simulink model "trabalho_funcionando"  (R2015a)
settings: Solver=ode23t  StartTime=0.0  StopTime=0.6  RelTol=1e-3
libraries: fl_lib x33, elec_lib x22, nesl_utility x22
Description:
  | Low-Noise Bipolar Transistor Voltage Amplifier
  | 
  | This example shows a typical low-noise audio amplifier circuit.
  | Resistor R2 provides negative feedback to stabilize the overall
  | amplifier gain, making it independent of transistor open-loop
  | forward transfer gain. Circuit gain is approximately defined by
  | (R1+R2)/R1 = 101. The simulation shows that it takes the circuit
  | a few seconds to settle to its steady operating point, and that the
  | output is initially clipped. Input u and output y are included to
  | support linearization.
  | 
  | If you have Simulink(R) Control Design(TM) installed, then to plot the
  | frequency response, select Analysis->Control Design-> Linear
  | Analysis to open the Linear Analysis Tool.
  | Before linearizing, you need to select the Solver Configuration block
  | option "Start simulation from steady state" to ensure that the model
  | is linearized about its nominal operating point. Change the Plot
  | Result to New Bode, and then click on Linearize. The linearization
  | points are defined by right-clicking on a Simulink(R) line, and
  | selecting Linearization Points.
  | If you look at the measurement block with input port V1, you will see
  | the linearization output symbol at the output of the PS-Simulink(R)
  | block. Similarly under the Source block you will see a linearization
  | input point symbol on the output of the Sine Wave block.
  | 
  | If you do not have Simulink Control Design, then you can
  | linearize the model between input port u and output port y
  | by typing:
  | 
  | [a,b,c,d] = linmod('elec_bipolar_low_noise_amp')
  | 
  | The frequency response can then be plotted using the
  | Control System Toolbox(TM) by typing:
  | 
  | bode(a,b,c,d)
  | 
  | 
  | 
  | Copyright 2008-2015 The MathWorks, Inc.
settings Model: CovSFcnEnable=off  Creator=MathWorks  LastModifiedBy=João Pedro
settings DataIOCC: SignalLoggingSaveFormat=ModelDataLogs
settings OptimizationCC: ExpressionDepthLimit=2147483647
settings DebuggingCC: UnderspecifiedInitializationDetection=Classic  MergeDetectMultiDrivingBlocksExec=none  FcnCallInpInsideContextMsg=UseLocalSettings  StateNameClashWarn=warning
settings GRTTargetCC: CombineOutputUpdateFcns=off  GRTInterface=on

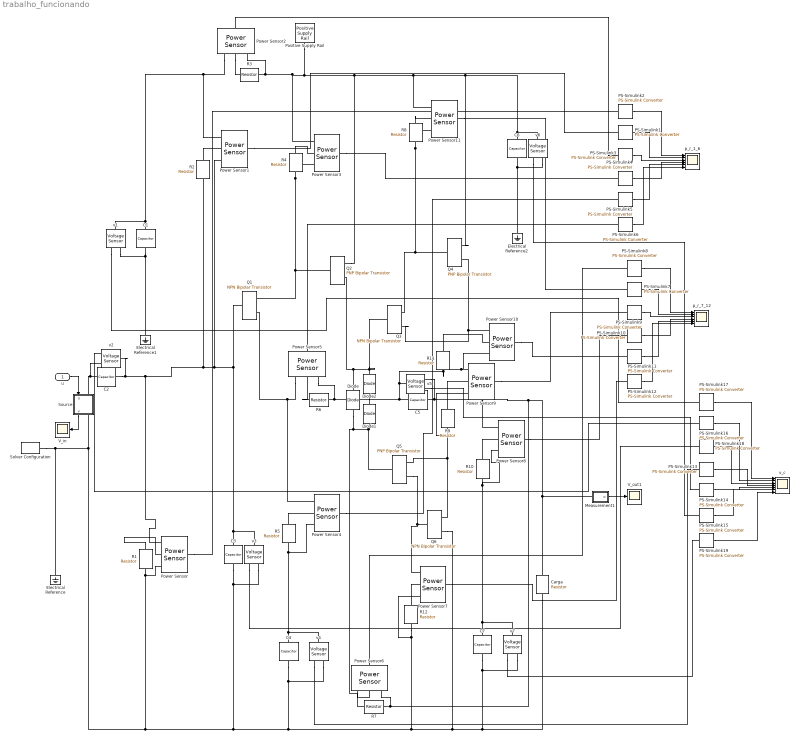
== system trabalho_funcionando ==
  u : Inport
  C1 : fl_lib/Electrical/Electrical Elements/Capacitor  c=2.2 uF  r=10 Ohm  g=0 1/Ohm  i_specify=off  i_priority=High  i=0 A  v_specify=off  v_priority=High  v=0 V  vc_specify=on  vc_priority=High  vc=0 V
  C2 : fl_lib/Electrical/Electrical Elements/Capacitor  c=1 uF  r=10 Ohm  g=0 1/Ohm  i_specify=off  i_priority=High  i=0 A  v_specify=off  v_priority=High  v=0 V  vc_specify=on  vc_priority=High  vc=0 V
  C3 : fl_lib/Electrical/Electrical Elements/Capacitor  c=47 pF  r=0.1 Ohm  g=0 1/Ohm  i_specify=off  i_priority=High  i=0 A  v_specify=off  v_priority=High  v=0 V  vc_specify=on  vc_priority=High  vc=0 V
  C4 : fl_lib/Electrical/Electrical Elements/Capacitor  c=47 uF  r=0.1 Ohm  g=0 1/Ohm  i_specify=off  i_priority=High  i=0 A  v_specify=off  v_priority=High  v=0 V  vc_specify=on  vc_priority=High  vc=0 V
  C5 : fl_lib/Electrical/Electrical Elements/Capacitor  c=2200 uF  r=0.1 Ohm  g=0 1/Ohm  i_specify=off  i_priority=High  i=0 A  v_specify=off  v_priority=High  v=0 V  vc_specify=on  vc_priority=High  vc=0 V
  C6 : fl_lib/Electrical/Electrical Elements/Capacitor  c=0.1 uF  r=10 Ohm  g=0 1/Ohm  i_specify=off  i_priority=High  i=0 A  v_specify=off  v_priority=High  v=0 V  vc_specify=on  vc_priority=High  vc=0 V
  C7 : fl_lib/Electrical/Electrical Elements/Capacitor  c=0.1 uF  r=10 Ohm  g=0 1/Ohm  i_specify=off  i_priority=High  i=0 A  v_specify=off  v_priority=High  v=0 V  vc_specify=on  vc_priority=High  vc=0 V
  Carga : fl_lib/Electrical/Electrical Elements/Resistor  R=4 Ohm  i_specify=off  i_priority=High  i=0 A  v_specify=off  v_priority=High  v=0 V
  Diode : elec_lib/Semiconductor Devices/Diode  ModelType=1  Vf=0.1 V  Ron=0.3 Ohm  Goff=1e-8 S  Rz=0.3 Ohm  Vz=50 V  C_PWL=5 pF  prmExp=1  I12=[ 0.0137 0.545 ] A  V12=[ 0.6 0.7 ] V  I1=0.0137 A  V1=0.6 V  RS=0.01 Ohm  IS=1e-12 A  Tmeas=25 C  ec=1  BV=Inf V  C_param=1  CJ0=5 pF  VJ=1 V  Mgrad=0.5  Vvec=[ 0.1 10 100 ] V  Cvec=[ 3.5 1 0.4 ] pF  FC=0.5  Q_param=1  Irrm=-7.15 A  iF=4 A  didt=-750 A/us  trr=115 ns  TT=50 ns  tau=100 ns  T_param=1  IS_T2=1.25e-7 A  I1_T2=0.245 A  V1_T2=0.5 V  Tmeas2=125 C  EG_param=1  EG=1.11 eV  XTI_param=1  XTI=3  dBVdT=0 V/K  Tdevice=25 C  Rth=[ 0 10 ] K/W  thermal_mass_parameterization=1  thermal_mass=[ 0 1 ] J/K  thermal_time_constant=[ 0 10 ] s  thermal_mass_initial_temperatures=[ 25 25 ] C
  Diode1 : elec_lib/Semiconductor Devices/Diode  ModelType=1  Vf=0.1 V  Ron=0.3 Ohm  Goff=1e-8 S  Rz=0.3 Ohm  Vz=50 V  C_PWL=5 pF  prmExp=1  I12=[ 0.0137 0.545 ] A  V12=[ 0.6 0.7 ] V  I1=0.0137 A  V1=0.6 V  RS=0.01 Ohm  IS=1e-12 A  Tmeas=25 C  ec=1  BV=Inf V  C_param=1  CJ0=5 pF  VJ=1 V  Mgrad=0.5  Vvec=[ 0.1 10 100 ] V  Cvec=[ 3.5 1 0.4 ] pF  FC=0.5  Q_param=1  Irrm=-7.15 A  iF=4 A  didt=-750 A/us  trr=115 ns  TT=50 ns  tau=100 ns  T_param=1  IS_T2=1.25e-7 A  I1_T2=0.245 A  V1_T2=0.5 V  Tmeas2=125 C  EG_param=1  EG=1.11 eV  XTI_param=1  XTI=3  dBVdT=0 V/K  Tdevice=25 C  Rth=[ 0 10 ] K/W  thermal_mass_parameterization=1  thermal_mass=[ 0 1 ] J/K  thermal_time_constant=[ 0 10 ] s  thermal_mass_initial_temperatures=[ 25 25 ] C
  Diode2 : elec_lib/Semiconductor Devices/Diode  ModelType=1  Vf=0.1 V  Ron=0.3 Ohm  Goff=1e-8 S  Rz=0.3 Ohm  Vz=50 V  C_PWL=5 pF  prmExp=1  I12=[ 0.0137 0.545 ] A  V12=[ 0.6 0.7 ] V  I1=0.0137 A  V1=0.6 V  RS=0.01 Ohm  IS=1e-12 A  Tmeas=25 C  ec=1  BV=Inf V  C_param=1  CJ0=5 pF  VJ=1 V  Mgrad=0.5  Vvec=[ 0.1 10 100 ] V  Cvec=[ 3.5 1 0.4 ] pF  FC=0.5  Q_param=1  Irrm=-7.15 A  iF=4 A  didt=-750 A/us  trr=115 ns  TT=50 ns  tau=100 ns  T_param=1  IS_T2=1.25e-7 A  I1_T2=0.245 A  V1_T2=0.5 V  Tmeas2=125 C  EG_param=1  EG=1.11 eV  XTI_param=1  XTI=3  dBVdT=0 V/K  Tdevice=25 C  Rth=[ 0 10 ] K/W  thermal_mass_parameterization=1  thermal_mass=[ 0 1 ] J/K  thermal_time_constant=[ 0 10 ] s  thermal_mass_initial_temperatures=[ 25 25 ] C
  Electrical Reference : fl_lib/Electrical/Electrical Elements/Electrical Reference
  Electrical Reference1 : fl_lib/Electrical/Electrical Elements/Electrical Reference
  Electrical Reference2 : fl_lib/Electrical/Electrical Elements/Electrical Reference
  Measurement1 : Subsystem
  PS-Simulink{1..19} (19 alike) : nesl_utility/PS-Simulink Converter  PhysicalDomain=network_engine_domain  SubClassName=ps_output  LeftPortType=input  RightPortType=output  PseudoPeriodic=off  Frequencies=[]  Unit=1  AffineConversion=off
  Positive Supply Rail : elec_lib/Sources/Positive Supply Rail  v0=54 V
  Power Sensor{,1..11} (12 alike) : elec_lib/Sensors/Power Sensor  measurement_type=1  averaging_period=1e-4 s
  Q1 : elec_lib/Semiconductor Devices/NPN Bipolar Transistor  parameterization=2  prmDatasheet=1  prmEquCoeff=1  BF=458.7  IS=4.68e-14 A  ec=1  VAF=52.64 V  hfe=520  hoe=5e-05 1/Ohm  Ic_h=100 mA  Vce_h=5 V  V1=0.55 V  I1=0.5 mA  BR=11.57  Tmeas=25 C  RC=1 Ohm  RE=0.26 Ohm  RB=1 Ohm  C_BC=4 pF  C_BE=4 pF  TF=0 us  TR=0 us  hfe_T2=125  XTB=0  V1_T2=0.45 V  I1_T2=0.5 mA  Tmeas2=125 C  EG=1.11 eV  XTI=3  TdeviceDatasheet=25 C  TdeviceEquCoeff=25 C  Rth=[ 0 10 ] K/W  thermal_mass_parameterization=1  thermal_mass=[ 0 1 ] J/K  thermal_time_constant=[ 0 10 ] s  thermal_mass_initial_temperatures=[ 25 25 ] C
  Q2 : elec_lib/Semiconductor Devices/PNP Bipolar Transistor  parameterization=2  prmDatasheet=1  prmEquCoeff=1  BF=449.8  IS=2.077e-13 A  ec=1  VAF=29 V  hfe=100  hoe=5e-5 1/Ohm  Ic_h=-1 mA  Vce_h=-5 V  V1=-0.55 V  I1=-0.5 mA  BR=20.92  Tmeas=25 C  RC=0.32 Ohm  RE=0.14 Ohm  RB=40 Ohm  C_BC=5 pF  C_BE=5 pF  TF=0 us  TR=0 us  hfe_T2=125  XTB=0  V1_T2=-0.45 V  I1_T2=-0.5 mA  Tmeas2=125 C  EG=1.11 eV  XTI=3  TdeviceDatasheet=25 C  TdeviceEquCoeff=25 C  Rth=[ 0 10 ] K/W  thermal_mass_parameterization=1  thermal_mass=[ 0 1 ] J/K  thermal_time_constant=[ 0 10 ] s  thermal_mass_initial_temperatures=[ 25 25 ] C
  Q3 : elec_lib/Semiconductor Devices/NPN Bipolar Transistor  parameterization=2  prmDatasheet=1  prmEquCoeff=1  BF=153.42  IS=800e-15 A  ec=1  VAF=4.8443 V  hfe=100  hoe=5e-05 1/Ohm  Ic_h=1 mA  Vce_h=5 V  V1=0.55 V  I1=0.5 mA  BR=39.462  Tmeas=25 C  RC=39.911 Ohm  RE=0.005 Ohm  RB=0.574 Ohm  C_BC=4 pF  C_BE=4 pF  TF=0 us  TR=0 us  hfe_T2=125  XTB=0  V1_T2=0.45 V  I1_T2=0.5 mA  Tmeas2=125 C  EG=1.11 eV  XTI=3  TdeviceDatasheet=25 C  TdeviceEquCoeff=25 C  Rth=[ 0 10 ] K/W  thermal_mass_parameterization=1  thermal_mass=[ 0 1 ] J/K  thermal_time_constant=[ 0 10 ] s  thermal_mass_initial_temperatures=[ 25 25 ] C
  Q4 : elec_lib/Semiconductor Devices/PNP Bipolar Transistor  parameterization=2  prmDatasheet=1  prmEquCoeff=1  BF=65.974  IS=7.899e-11 A  ec=1  VAF=10.7084 V  hfe=100  hoe=5e-5 1/Ohm  Ic_h=-1 mA  Vce_h=-5 V  V1=-0.55 V  I1=-0.5 mA  BR=1.9619  Tmeas=25 C  RC=0.12 Ohm  RE=1e-4 Ohm  RB=2.355 Ohm  C_BC=5 pF  C_BE=5 pF  TF=0 us  TR=0 us  hfe_T2=125  XTB=0  V1_T2=-0.45 V  I1_T2=-0.5 mA  Tmeas2=125 C  EG=1.11 eV  XTI=3  TdeviceDatasheet=25 C  TdeviceEquCoeff=25 C  Rth=[ 0 10 ] K/W  thermal_mass_parameterization=1  thermal_mass=[ 0 1 ] J/K  thermal_time_constant=[ 0 10 ] s  thermal_mass_initial_temperatures=[ 25 25 ] C
  Q5 : elec_lib/Semiconductor Devices/PNP Bipolar Transistor  parameterization=2  prmDatasheet=1  prmEquCoeff=1  BF=222.84  IS=400e-15 A  ec=1  VAF=30.600 V  hfe=100  hoe=5e-5 1/Ohm  Ic_h=-1 mA  Vce_h=-5 V  V1=-0.55 V  I1=-0.5 mA  BR=10.181  Tmeas=25 C  RC=0.27337 Ohm  RE=40e-3 Ohm  RB=1.7344 Ohm  C_BC=5 pF  C_BE=5 pF  TF=0 us  TR=0 us  hfe_T2=125  XTB=0  V1_T2=-0.45 V  I1_T2=-0.5 mA  Tmeas2=125 C  EG=1.11 eV  XTI=3  TdeviceDatasheet=25 C  TdeviceEquCoeff=25 C  Rth=[ 0 10 ] K/W  thermal_mass_parameterization=1  thermal_mass=[ 0 1 ] J/K  thermal_time_constant=[ 0 10 ] s  thermal_mass_initial_temperatures=[ 25 25 ] C
  Q6 : elec_lib/Semiconductor Devices/NPN Bipolar Transistor  parameterization=2  prmDatasheet=1  prmEquCoeff=1  BF=73  IS=2.37e-8 A  ec=1  VAF=100 V  hfe=100  hoe=5e-05 1/Ohm  Ic_h=1 mA  Vce_h=5 V  V1=0.55 V  I1=0.5 mA  BR=2.66  Tmeas=25 C  RC=0.0856 Ohm  RE=0.000856 Ohm  RB=0.81 Ohm  C_BC=4 pF  C_BE=4 pF  TF=0 us  TR=0 us  hfe_T2=125  XTB=0  V1_T2=0.45 V  I1_T2=0.5 mA  Tmeas2=125 C  EG=1.11 eV  XTI=3  TdeviceDatasheet=25 C  TdeviceEquCoeff=25 C  Rth=[ 0 10 ] K/W  thermal_mass_parameterization=1  thermal_mass=[ 0 1 ] J/K  thermal_time_constant=[ 0 10 ] s  thermal_mass_initial_temperatures=[ 25 25 ] C
  R1 : fl_lib/Electrical/Electrical Elements/Resistor  R=220 kOhm  i_specify=off  i_priority=High  i=0 A  v_specify=off  v_priority=High  v=0 V
  R10 : fl_lib/Electrical/Electrical Elements/Resistor  R=10 Ohm  i_specify=off  i_priority=High  i=0 A  v_specify=off  v_priority=High  v=0 V
  R11 : fl_lib/Electrical/Electrical Elements/Resistor  R=0.47 Ohm  i_specify=off  i_priority=High  i=0 A  v_specify=off  v_priority=High  v=0 V
  R12 : fl_lib/Electrical/Electrical Elements/Resistor  R=180 Ohm  i_specify=off  i_priority=High  i=0 A  v_specify=off  v_priority=High  v=0 V
  R2 : fl_lib/Electrical/Electrical Elements/Resistor  R=150 kOhm  i_specify=off  i_priority=High  i=0 A  v_specify=off  v_priority=High  v=0 V
  R3 : fl_lib/Electrical/Electrical Elements/Resistor  R=47 kOhm  i_specify=off  i_priority=High  i=0 A  v_specify=off  v_priority=High  v=0 V
  R4 : fl_lib/Electrical/Electrical Elements/Resistor  R=5.6 kOhm  i_specify=off  i_priority=High  i=0 A  v_specify=off  v_priority=High  v=0 V
  R5 : fl_lib/Electrical/Electrical Elements/Resistor  R=270 Ohm  i_specify=off  i_priority=High  i=0 A  v_specify=off  v_priority=High  v=0 V
  R6 : fl_lib/Electrical/Electrical Elements/Resistor  R=10 kOhm  i_specify=off  i_priority=High  i=0 A  v_specify=off  v_priority=High  v=0 V
  R7 : fl_lib/Electrical/Electrical Elements/Resistor  R=8.2 kOhm  i_specify=off  i_priority=High  i=0 A  v_specify=off  v_priority=High  v=0 V
  R8 : fl_lib/Electrical/Electrical Elements/Resistor  R=180 Ohm  i_specify=off  i_priority=High  i=0 A  v_specify=off  v_priority=High  v=0 V
  R9 : fl_lib/Electrical/Electrical Elements/Resistor  R=0.39 Ohm  i_specify=off  i_priority=High  i=0 A  v_specify=off  v_priority=High  v=0 V
  Solver Configuration : nesl_utility/Solver Configuration  PhysicalDomain=network_engine_domain  SubClassName=solver  LeftPortType=input  RightPortType=generic  Accelerate=off  Tones=[]  Harmonics=[]  SimulateNoise=off  Profile=off  UseLocalSampling=off  EnableSwitchedLinearOptims=on  FrequencyDomain=off  UseCCode=off  RelTol=0.001  AbsTol=1e-06  MinStep=1e-09  ToWorkspace=off  RevertToSquareIcSolve=off  NumHomotopyIterations=100  DoDC=off  ResidualTolerance=1e-9  UseLocalSolver=off  LocalSolverChoice=NE_BACKWARD_EULER_ADVANCER  LocalSolverSampleTime=1e-5  DoFixedCost=off  MaxNonlinIter=2  MaxModeIter=2  LinearAlgebra=Sparse  DelaysMemoryBudget=1024  AutomaticFiltering=on  FilteringTimeConstant=0.001
  Source : Subsystem
  V_in : Scope
      settings: TimeRange=0.01  YMin=-0.1  YMax=0.1
  V_out1 : Scope
      settings: TimeRange=0.01  YMin=-10  YMax=10  SaveName=ScopeData2
  p_r_1_6 : Scope  NumInputPorts=6
      settings: TimeRange=0.01  YMin=-10~-5~-5~-5~-5~-5  YMax=10~5~5~5~5~5
  p_r_7_12 : Scope  NumInputPorts=6
      settings: TimeRange=0.01  YMin=-10~-5~-5~-5~-5~-5  YMax=10~5~5~5~5~5  SaveName=ScopeData3
  v{1..7} (7 alike) : fl_lib/Electrical/Electrical Sensors/Voltage Sensor
  v_c : Scope  NumInputPorts=7
      settings: TimeRange=0.01  YMin=-10~-5~-5~-5~-5~-5~-5  YMax=10~5~5~5~5~5~5  SaveName=ScopeData4
  wires:
  Source/1(v) -> V_in/1
  u/1 -> Source/1(u)
  Measurement1/1(o) -> V_out1/1
  PS-Simulink2/1 -> p_r_1_6/1
  PS-Simulink1/1 -> p_r_1_6/2
  PS-Simulink3/1 -> p_r_1_6/3
  PS-Simulink4/1 -> p_r_1_6/4
  PS-Simulink5/1 -> p_r_1_6/5
  PS-Simulink6/1 -> p_r_1_6/6
  PS-Simulink8/1 -> p_r_7_12/1
  PS-Simulink7/1 -> p_r_7_12/2
  PS-Simulink9/1 -> p_r_7_12/3
  PS-Simulink10/1 -> p_r_7_12/4
  PS-Simulink11/1 -> p_r_7_12/5
  PS-Simulink12/1 -> p_r_7_12/6
  PS-Simulink17/1 -> v_c/1
  PS-Simulink16/1 -> v_c/2
  PS-Simulink18/1 -> v_c/3
  PS-Simulink13/1 -> v_c/4
  PS-Simulink14/1 -> v_c/5
  PS-Simulink15/1 -> v_c/6
  PS-Simulink19/1 -> v_c/7
  connections:
  Solver Configuration/RConn1 -- Electrical Reference/LConn1 -- Power Sensor/LConn3 -- R1/RConn1 -- v3/RConn2 -- C3/RConn1 -- v4/RConn2 -- C4/RConn1 -- Power Sensor7/LConn3 -- R12/LConn1 -- v7/RConn2 -- C7/RConn1 -- Carga/LConn1 -- Q6/RConn2 -- Source/RConn1
  Q2/LConn1 -- Power Sensor3/LConn3 -- R4/LConn1 -- Q1/RConn1
  Source/LConn1 -- v2/RConn2 -- C2/RConn1
  C1/RConn1 -- v1/RConn2 -- Electrical Reference1/LConn1
  C1/LConn1 -- v1/LConn1 -- Power Sensor2/LConn1 -- Power Sensor1/LConn1
  C3/LConn1 -- v3/LConn1 -- Power Sensor1/LConn3 -- v2/LConn1 -- C2/LConn1 -- Power Sensor/LConn1 -- R2/LConn1 -- Q1/LConn1
  R3/LConn1 -- Power Sensor3/LConn1 -- Power Sensor11/LConn1 -- v6/LConn1 -- C6/LConn1 -- Q4/RConn1 -- Q2/RConn1 -- Positive Supply Rail/RConn1 -- Power Sensor2/LConn3
  Power Sensor4/LConn1 -- Q1/RConn2 -- Power Sensor5/LConn1
  C4/LConn1 -- v4/LConn1 -- Power Sensor4/LConn3 -- R5/LConn1
  Q3/LConn1 -- Diode2/RConn1 -- Diode/LConn1 -- Q2/RConn2
  Q5/RConn2 -- Power Sensor7/LConn1 -- Q6/LConn1
  Q6/RConn1 -- Power Sensor9/LConn3 -- R9/LConn1 -- Q5/RConn1
  R6/RConn1 -- Power Sensor5/LConn3 -- C5/LConn1 -- Power Sensor10/LConn3 -- Power Sensor9/LConn1 -- R11/LConn1 -- v5/LConn1
  Power Sensor8/LConn2 -- R10/RConn1
  Q4/LConn1 -- Power Sensor11/LConn3 -- R8/LConn1 -- Q3/RConn1
  Q3/RConn2 -- Q4/RConn2 -- Power Sensor10/LConn1
  Electrical Reference2/LConn1 -- v6/RConn2 -- C6/RConn1
  C7/LConn1 -- v7/LConn1 -- Power Sensor8/LConn3 -- R10/LConn1
  Diode1/LConn1 -- Power Sensor6/LConn1 -- Diode/RConn1 -- Q5/LConn1
  Diode2/LConn1 -- Diode1/RConn1
  Power Sensor/LConn2 -- R1/LConn1
  Power Sensor1/LConn2 -- R2/RConn1
  Power Sensor2/LConn2 -- R3/RConn1
  Power Sensor3/LConn2 -- R4/RConn1
  Power Sensor4/LConn2 -- R5/RConn1
  R6/LConn1 -- Power Sensor5/LConn2
  Power Sensor/RConn1 -- PS-Simulink2/LConn1
  Power Sensor1/RConn1 -- PS-Simulink1/LConn1
  Power Sensor2/RConn1 -- PS-Simulink3/LConn1
  Power Sensor3/RConn1 -- PS-Simulink4/LConn1
  Power Sensor4/RConn1 -- PS-Simulink5/LConn1
  Power Sensor5/RConn1 -- PS-Simulink6/LConn1
  R7/LConn1 -- Power Sensor6/LConn2
  Power Sensor7/LConn2 -- R12/RConn1
  C5/RConn1 -- v5/RConn2 -- Power Sensor8/LConn1 -- Power Sensor6/LConn3 -- R7/RConn1 -- Carga/RConn1 -- Measurement1/LConn1
  R9/RConn1 -- Power Sensor9/LConn2
  Power Sensor10/LConn2 -- R11/RConn1
  R8/RConn1 -- Power Sensor11/LConn2
  Power Sensor6/RConn1 -- PS-Simulink8/LConn1
  Power Sensor11/RConn1 -- PS-Simulink7/LConn1
  Power Sensor9/RConn1 -- PS-Simulink9/LConn1
  Power Sensor7/RConn1 -- PS-Simulink12/LConn1
  Power Sensor8/RConn1 -- PS-Simulink10/LConn1
  Power Sensor10/RConn1 -- PS-Simulink11/LConn1
  v1/RConn1 -- PS-Simulink17/LConn1
  v2/RConn1 -- PS-Simulink16/LConn1
  v3/RConn1 -- PS-Simulink18/LConn1
  v4/RConn1 -- PS-Simulink13/LConn1
  v5/RConn1 -- PS-Simulink14/LConn1
  v7/RConn1 -- PS-Simulink19/LConn1
  v6/RConn1 -- PS-Simulink15/LConn1

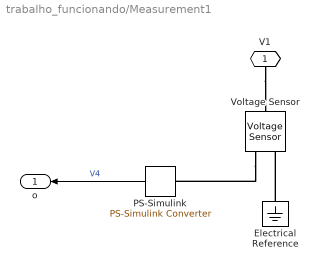
== system trabalho_funcionando/Measurement1 ==
  Electrical Reference : fl_lib/Electrical/Electrical Elements/Electrical Reference
  PS-Simulink : nesl_utility/PS-Simulink Converter  PhysicalDomain=network_engine_domain  SubClassName=ps_output  LeftPortType=input  RightPortType=output  PseudoPeriodic=off  Frequencies=[]  Unit=1  AffineConversion=off
  Voltage Sensor : fl_lib/Electrical/Electrical Sensors/Voltage Sensor
  V1 : PMIOPort  Port=1  Side=Left
  o : Outport
  wires:
  PS-Simulink/1 -> o/1  "V4"
  connections:
  Electrical Reference/LConn1 -- Voltage Sensor/RConn2
  V1/RConn1 -- Voltage Sensor/LConn1
  Voltage Sensor/RConn1 -- PS-Simulink/LConn1

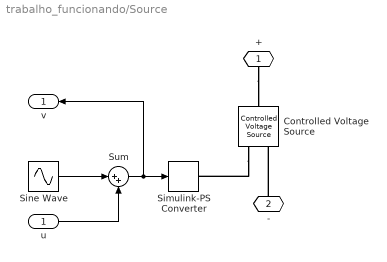
== system trabalho_funcionando/Source ==
  u : Inport
  Controlled Voltage Source : fl_lib/Electrical/Electrical Sources/Controlled Voltage Source
  Simulink-PS Converter : nesl_utility/Simulink-PS Converter  PhysicalDomain=network_engine_domain  SubClassName=ps_input  LeftPortType=input  RightPortType=output  PseudoPeriodic=off  Frequencies=[]  NoiseDistribution=none  NoiseParameters=[]  Unit=V  AffineConversion=off  InputFiltering=off  SimscapeFilterOrder=1  InputFilterTimeConstant=.001  UdotUserProvided=0
  Sine Wave : Sin  Amplitude=0.25  Frequency=2*pi*1000  SampleTime=0
  Sum : Sum  Inputs=|++
  + : PMIOPort  Port=1  Side=Left
  - : PMIOPort  Port=2  Side=Right
  v : Outport
  wires:
  u/1 -> Sum/2
  Sum/1 -> Simulink-PS Converter/1, v/1
  Sine Wave/1 -> Sum/1
  connections:
  Controlled Voltage Source/RConn1 -- Simulink-PS Converter/RConn1
  -/RConn1 -- Controlled Voltage Source/RConn2
  +/RConn1 -- Controlled Voltage Source/LConn1
